simulink model "zumobot_host"  (R2014b)
settings: Solver=FixedStepDiscrete  StartTime=0.0  StopTime=inf  RelTol=1e-3
undefined symbols (not defined in the file or in its folder): IsPositionTracked, IsSkeletonTracked, JointDepthIndices, JointImageIndices, JointTrackingState, JointWorldCoordinates, none, PositionDepthIndices, PositionImageIndices, PositionWorldCoordinates, SegmentationData, SkeletonTrackingID, videoinput
libraries: visiontextngfix x1, imaqlib x1, arduinolib x1, visionsinks x1
settings Model: Creator=sandip  LastModifiedBy=sandip

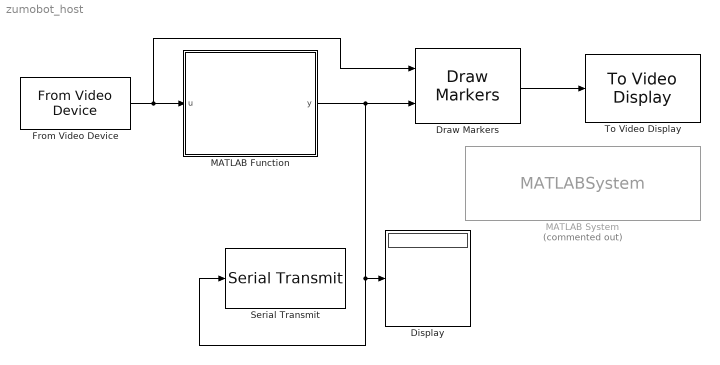
== system zumobot_host ==
  Display : Display
  Draw Markers : visiontextngfix/Draw Markers  shape=X-mark  size=5  fill=off  fillClrSource=Specify via dialog  display=User-specified value  intensity=200  color=[255 0 0]  opacity=0.6  viewport=Entire image  antialiasing=off  inType=Obsolete  imagePorts=One multidimensional signal  prodOutputMode=Binary point scaling  prodOutputWordLength=32  prodOutputFracLength=14  memoryMode=Specify word length  memoryWordLength=16  memoryFracLength=15  roundingMode=Floor  overflowMode=off
  From Video Device : imaqlib/From Video Device  DeviceMenu=winvideo 2 (Microsoft LifeCam Cinema)  Device=winvideo 2 (Microsoft LifeCam Cinema)  ObjConstructor=videoinput('winvideo', 2)  VideoFormatMenu=YUY2_800x600  VideoFormat=YUY2_800x600  VideoSource=input1  ROIPosition=[0 0 600 800]  EnableHWTrigger=off  TriggerConfiguration=none/none  SampleTime=1/10  OutputPortsMode=One multidimensional signal  DataType=single  CanDoHWTrigger=no  ReturnedColorSpace=rgb  BlockHandle=1921.0006  ROIWidth=800  ROIHeight=600  ROIColumn=0  ROIRow=0  EngXMLPath=C:\Program Files\MATLAB\R2014b\toolbox\imaq\imaq\private  DevXMLPath=C:\MATLAB\SupportPackages\R2014b\osgenericvideointerface\toolbox\imaq\supportpackages\genericvideo\adaptor\win64  EngLibPath=C:\Program Files\MATLAB\R2014b\toolbox\imaq\imaqblks\imaqmex\win64  ColorSpace=rgb  BayerSensorAlignment=grbg  AllMetadata=IsPositionTracked;IsSkeletonTracked;JointDepthIndices;JointImageIndices;JointTrackingState;JointWorldCoordinates;PositionDepthIndices;PositionImageIndices;PositionWorldCoordinates;SegmentationData;SkeletonTrackingID
  MATLAB Function : MATLAB Function  TreatAsAtomicUnit=on
  MATLAB System : MATLABSystem  Commented=on  DialogController=sysobjdialog.BlockDynDialog  System=vision.PointTracker  MaxBidirectionalError=inf  BlockSize=[ 31, 31 ]  NumPyramidLevels=3  MaxIterations=30
      mask Type: vision.PointTracker
      mask Display:
      | disp('PointTracker');
      | port_label('input',1,'I');
      | port_label('output',1,'points');
      | port_label('output',2,'pointValidity');
      | port_label('output',3,'scores');
  Serial Transmit : arduinolib/Serial Transmit  portNumber=0  blockPlatform=arduino
  To Video Display : visionsinks/To Video Display  inputType=Obsolete  imagePorts=One multidimensional signal  OutputDevice=On-screen video monitor  fullScreen=off  videoWindowX=938  videoWindowY=227  saveWindowSize=off  videoWindowWidth=800  videoWindowHeight=600  dataOrg=Column-major  openAtMdlStart=on  isWindowOpen=on  inputColorFormat=RGB
  wires:
  From Video Device/1 -> Draw Markers/1, MATLAB Function/1(u)
  MATLAB Function/1(y) -> Draw Markers/2, Serial Transmit/1, Display/1
  Draw Markers/1 -> To Video Display/1

== matlab function zumobot_host/MATLAB Function ==
  data: u input; y output
function y = fcn(u)
%#codegen
y = ones([1,2],'uint16');
coder.extrinsic('detectZumoAndSphero');
[y, ~] = detectZumoAndSphero(u);

%coder.extrinsic('vision.PointTracker');
